simulink model "Parallel"  (R2020b)
settings: Solver=ode4  StartTime=0  StopTime=endtime  MaxStep=0.05  RelTol=1e-5
values from neighbouring files (symbols this model uses):
  Av = 1.545*1.805    (= 2.788725)    [InitiateParallel.m]
  Cd = 0.3    [InitiateParallel.m]
  Cr = 0.0032    [InitiateParallel.m]
  DCT = 1    [InitiateParallel.m]
  Density = (85*19.6e6 + 15*32e6)/100    (= 21460000)    [InitiateParallel.m]
  Eta_gen = 0.6    [InitiateParallel.m]
  EtaEM = Eta    [CreateEMmap.m]
  EtaGEAR = 0.97    [InitiateParallel.m]
  EtaICE = EtaICE_HeavyDIESEL    [InitiateParallel.m]
  EtaPE = 0.98    [InitiateParallel.m]
  grav = 9.81    [InitiateParallel.m]
  ksoc = max(Wbatt)/400/Tau_charge    [InitiateParallel.m]
  ksoc_vect = ksoc*tan(pi/2.05*[-1:1/15:1])*2    [InitiateParallel.m]
  Mv = 40000    [InitiateParallel.m]
  Number_of_gears = 12    [InitiateParallel.m]
  Paux = 3000    [InitiateParallel.m]
  Pem_max = 300000    [InitiateParallel.m]    (also in ParallelBatch_2D.m = EMpower_vector(loop2))
  Pice_max = 300000    [InitiateParallel.m]
  PtoT = zeros(length(P),4)    [CreateICEmap.m]
  rho_air = 1.2    [InitiateParallel.m]
  rw = 0.506    [InitiateParallel.m]
  SOC_batt_ref_value = 70    [InitiateParallel.m]
  SOC_batt_start_value = 100    [InitiateParallel.m]    (also in ParallelBatch_1D.m = SOC(length(SOC(:,1)),2))
  SOC_tract_max = 98    [InitiateParallel.m]
  SOC_tract_min = 12    [InitiateParallel.m]
  Tau_charge = 2    [InitiateParallel.m]
  Tem = Tem_max.*Tref/max(Tref)    [CreateEMmap.m]
  Tem_lim = min([Tem_max*ones(1,length(Wem)); Pem_max./Wem])    [CreateEMmap.m]
  Tem_max = Pem_max/(wice_max/fwr)    (= 2406.42273955)    [InitiateParallel.m]
  Tice_max = Pice_max/(wice_max*row/(length(EtaICE)-1))    [InitiateParallel.m]
  utvx_max = wice_max/((vmax/5)/rw)    (= 26.4940980453)    [InitiateParallel.m]
  Utvx_vect = zeros(1,Number_of_gears+1)    [InitiateParallel.m]
  Wbatt = 8.9*3.6e6    (= 32040000)    [InitiateParallel.m]
  Wem = wem_max.*w/max(w)    [CreateEMmap.m]
  wem_max = wice_max    (= 261.799387799)    [InitiateParallel.m]
  wice_max = 2500*2*pi/60    (= 261.799387799)    [InitiateParallel.m]
  wice_min = 700*2*pi/60    (= 73.3038285838)    [InitiateParallel.m]
undefined symbols (not defined in the file or in its folder): EtaBATT, FuelConsICE, Pbatt, Pbatt_max_new, Pice_max_parallel, Tice, Tlim_ice, Wice
libraries: simulink_need_slupdate x1, simulink x1
(part 1 of 2)
settings Model: ExtModeTrigMode=oneshot  ExtModeArmWhenConnect=off  Creator=Mats  LastModifiedBy=ielmats
settings DataIOCC: SaveFormat=Array  SignalLoggingSaveFormat=ModelDataLogs  ReturnWorkspaceOutputs=off  SignalLoggingName=sigsOut
settings OptimizationCC: BlockReduction=off  BooleanDataType=off  ExpressionDepthLimit=2147483647  InitFltsAndDblsToZero=on  LifeSpan=inf
settings DebuggingCC: ConsistencyChecking=warning  SaveWithParameterizedLinksMsg=none  UnderspecifiedInitializationDetection=Classic  MergeDetectMultiDrivingBlocksExec=none  SignalResolutionControl=TryResolveAllWithWarning  MultiTaskDSMMsg=warning  MultiTaskCondExecSysMsg=none  UnnecessaryDatatypeConvMsg=warning  FcnCallInpInsideContextMsg=warning  UnconnectedInputMsg=none  UnconnectedOutputMsg=none  UnconnectedLineMsg=none  StateNameClashWarn=warning  SFUnexpectedBacktrackingDiag=warning  SFNoUnconditionalDefaultTransitionDiag=warning  ArithmeticOperatorsInVariantConditions=warning
settings HardwareCC: ProdBitPerPointer=32  ProdBitPerSizeT=32  ProdBitPerPtrDiffT=32  ProdLargestAtomicFloat=None  ProdIntDivRoundTo=Undefined  ProdEndianess=Unspecified  ProdWordSize=32  ProdHWDeviceType=32-bit Generic  TargetHWDeviceType=32-bit Generic  TargetUnknown=on  ProdEqTarget=off
settings ModelReferenceCC: PropagateSignalLabelsOutOfModel=off
settings SFSimCC: SimUseLocalCustomCode=off  CustomCodeUndefinedFunction=UseInterfaceOnly
settings RTWCC: RTWUseLocalCustomCode=off
settings CodeAppCC: StateflowObjectComments=on
settings GRTTargetCC: TargetFcnLib=ansi_tfl_tmw.mat  TargetLangStandard=C89/C90 (ANSI)  CombineOutputUpdateFcns=off  GRTInterface=on
settings ConfigComp: CovMetricSettings=dw  CovSaveCumulativeToWorkspaceVar=on  CovSaveSingleToWorkspaceVar=on  CovExternalEMLEnable=off

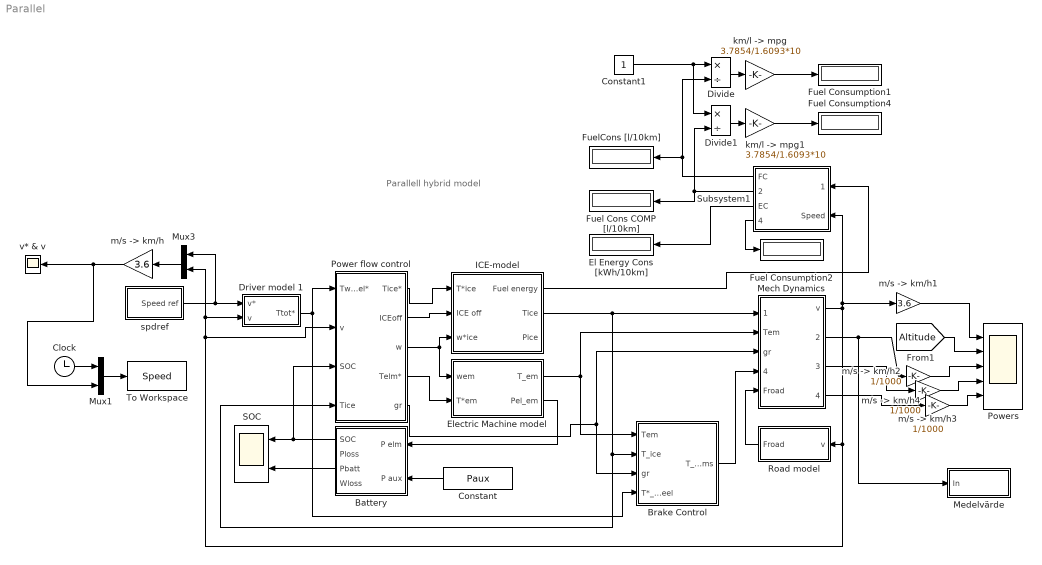
== system Parallel ==
  note: Parallell hybrid model
  Battery : Subsystem
  Brake Control : Subsystem
  Clock : Clock
  Constant : Constant  Value=Paux
  Constant1 : Constant
  Divide : Product  Inputs=*/
  Divide1 : Product  Inputs=*/
  Driver model 1 : Subsystem  mask{Mv=Mv, rw=rw, Pmax=Pice_max+Pem_max}
      mask prompts: Mv "Vehicle Mass"; rw "Wheel Radius"; Pmax "Max Wheel Power"
      mask init:
      | Ti = 2 + 1*(Mv-1000)/19000;
      | Kv=4*Mv/Ti;
  El Energy Cons [kWh/10km] : Display
  Electric Machine model : Subsystem
  Fuel Cons COMP [l/10km] : Display
  Fuel Consumption1 : Display
  Fuel Consumption2 : Display
  Fuel Consumption4 : Display
  FuelCons [l/10km] : Display
  ICE-model : Subsystem
  Mech Dynamics : Subsystem
  Medelvärde : Subsystem
  Mux1 : Mux  Inputs=2
  Mux3 : Mux  Inputs=2
  Power flow control : Subsystem
  Powers : Scope  NumInputPorts=5
  Road model : Subsystem
  SOC : Scope  NumInputPorts=2
  Subsystem1 : Subsystem
  To Workspace : ToWorkspace  VariableName=Speed  SampleTime=-1
  "km/l -> mpg" : Gain  Gain=3.7854/1.6093*10  SaturateOnIntegerOverflow=on  OutDataTypeStr=Inherit: Same as input  ParamDataTypeStr=Inherit: Same as input
  "km/l -> mpg1" : Gain  Gain=3.7854/1.6093*10  SaturateOnIntegerOverflow=on  OutDataTypeStr=Inherit: Same as input  ParamDataTypeStr=Inherit: Same as input
  "m/s -> km/h" : Gain  Gain=3.6  SaturateOnIntegerOverflow=on  OutDataTypeStr=Inherit: Same as input  ParamDataTypeStr=Inherit: Same as input
  "m/s -> km/h1" : Gain  Gain=3.6  SaturateOnIntegerOverflow=on  OutDataTypeStr=Inherit: Same as input  ParamDataTypeStr=Inherit: Same as input
  "m/s -> km/h2" : Gain  Gain=1/1000  SaturateOnIntegerOverflow=on  OutDataTypeStr=Inherit: Same as input  ParamDataTypeStr=Inherit: Same as input
  "m/s -> km/h3" : Gain  Gain=1/1000  SaturateOnIntegerOverflow=on  OutDataTypeStr=Inherit: Same as input  ParamDataTypeStr=Inherit: Same as input
  "m/s -> km/h4" : Gain  Gain=1/1000  SaturateOnIntegerOverflow=on  OutDataTypeStr=Inherit: Same as input  ParamDataTypeStr=Inherit: Same as input
  spdref : Subsystem
  v* & v : Scope
  wires:
  Power flow control/3(w) -> ICE-model/3(w*ice), Electric Machine model/1(wem)
  Constant/1 -> Battery/2(P aux)
  spdref/1(Speed ref) -> Driver model 1/1(v*), Mux3/1
  Driver model 1/1(Ttot*) -> Brake Control/4(T*_wheel), Power flow control/1(Twheel*)
  Mux3/1 -> "m/s -> km/h"/1
  Power flow control/5(gr) -> Brake Control/3(gr), Mech Dynamics/3(gr)
  Power flow control/4(Telm*) -> Electric Machine model/2(T*em)
  Power flow control/1(Tice*) -> ICE-model/1(T*ice)
  Mech Dynamics/1(v) -> Subsystem1/2(Speed), "m/s -> km/h1"/1, Driver model 1/2(v), Mux3/2, Power flow control/2(v), Road model/1("v ")
  Electric Machine model/1(T_em) -> Mech Dynamics/2(Tem), Brake Control/1(Tem)
  Electric Machine model/2(Pel_em) -> Battery/1(P elm)
  "m/s -> km/h"/1 -> Mux1/2, v* & v/1
  Battery/1(SOC) -> SOC/1, Power flow control/3(SOC)
  Power flow control/2(ICEoff) -> ICE-model/2(ICE off)
  Battery/3(Pbatt) -> SOC/2
  ICE-model/2(Tice) -> Power flow control/4(Tice), Brake Control/2(T_ice), Mech Dynamics/1(Tdrive)
  ICE-model/1(Fuel energy) -> Subsystem1/1(Fuel energy)
  [Altitude] -> Powers/2
  Mech Dynamics/2(Ptraction) -> Medelvärde/1(In), "m/s -> km/h2"/1
  Mech Dynamics/3(Pfriction) -> "m/s -> km/h3"/1
  Mech Dynamics/4(Pbrake) -> "m/s -> km/h4"/1
  "m/s -> km/h1"/1 -> Powers/1
  "m/s -> km/h2"/1 -> Powers/3
  "m/s -> km/h3"/1 -> Powers/4
  "m/s -> km/h4"/1 -> Powers/5
  Brake Control/1(T_broms) -> Mech Dynamics/4(Tbrake)
  Road model/1(Froad) -> Mech Dynamics/5(Froad)
  Subsystem1/4(dist (mil)) -> Fuel Consumption2/1
  Clock/1 -> Mux1/1
  Mux1/1 -> To Workspace/1
  Constant1/1 -> Divide1/1, Divide/1
  Divide/1 -> "km/l -> mpg"/1
  Subsystem1/1(FC) -> FuelCons [l/10km]/1, Divide/2
  Subsystem1/2(FCcomp) -> Divide1/2, Fuel Cons COMP [l/10km]/1
  Divide1/1 -> "km/l -> mpg1"/1
  "km/l -> mpg"/1 -> Fuel Consumption1/1
  "km/l -> mpg1"/1 -> Fuel Consumption4/1
  Subsystem1/3(EC) -> El Energy Cons [kWh/10km]/1

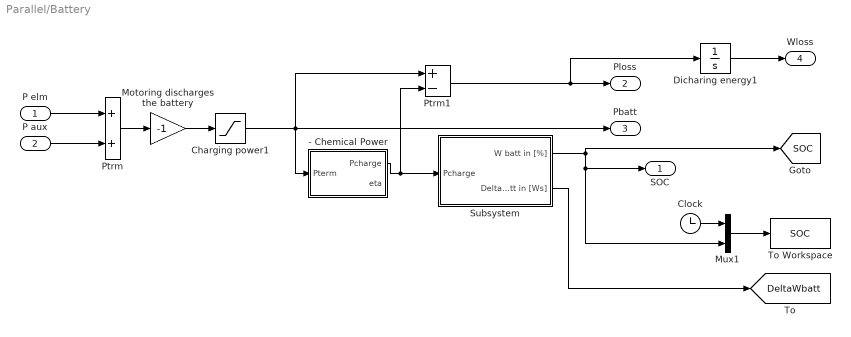
== system Parallel/Battery ==
  P elm : Inport
  P aux : Inport  Port=2
  - Chemical Power : Subsystem
  Charging power1 : Saturate  UpperLimit=Pbatt_max_new  LowerLimit=-Pbatt_max_new
  Clock : Clock
  Dicharing energy1 : Integrator  UpperSaturationLimit=-1
  Motoring discharges the battery : Gain  Gain=-1  SaturateOnIntegerOverflow=on  OutDataTypeStr=Inherit: Same as input  ParamDataTypeStr=Inherit: Same as input
  Mux1 : Mux  Inputs=2
  Ptrm : Sum  InputSameDT=on  SaturateOnIntegerOverflow=on  OutDataTypeStr=Inherit: Same as first input
  Ptrm1 : Sum  Inputs=+-  InputSameDT=on  SaturateOnIntegerOverflow=on  OutDataTypeStr=Inherit: Same as first input
  Subsystem : Subsystem
  To Workspace : ToWorkspace  VariableName=SOC  SampleTime=-1
  SOC : Outport  InitialOutput=0  VectorParamsAs1DForOutWhenUnconnected=off
  Ploss : Outport  Port=2  InitialOutput=0  VectorParamsAs1DForOutWhenUnconnected=off
  Pbatt : Outport  Port=3  InitialOutput=0  VectorParamsAs1DForOutWhenUnconnected=off
  Wloss : Outport  Port=4  InitialOutput=0  VectorParamsAs1DForOutWhenUnconnected=off
  tag scope: DeltaWbatt=global, SOC=global
  wires:
  P elm/1 -> Ptrm/1
  Ptrm/1 -> Motoring discharges the battery/1
  - Chemical Power/1(Pcharge) -> Ptrm1/2, Subsystem/1("Pcharge ")
  Ptrm1/1 -> Ploss/1, Dicharing energy1/1
  Motoring discharges the battery/1 -> Charging power1/1
  P aux/1 -> Ptrm/2
  Dicharing energy1/1 -> Wloss/1
  Charging power1/1 -> - Chemical Power/1(Pterm), Pbatt/1, Ptrm1/1
  Subsystem/1(W batt in [%]) -> Mux1/2, SOC/1, [SOC]
  Clock/1 -> Mux1/1
  Mux1/1 -> To Workspace/1
  Subsystem/2(DeltaWbatt in [Ws]) -> [DeltaWbatt]

== system Parallel/Brake Control ==
  note: If the drive train is not able
      | to supply the braking force, then
      | the friction brakes are used.
  Tem : Inport
  T_ice : Inport  Port=2
  gr : Inport  Port=3
  T*_wheel : Inport  Port=4
  -> hjulmoment : Product  InputSameDT=on  SaturateOnIntegerOverflow=on  OutDataTypeStr=Inherit: Same as first input
  Endast negativa bromsmoment1 : Saturate  UpperLimit=0  LowerLimit=-inf
  Mux : Mux  Inputs=2
  Scope : Scope
  Sum1 : Sum  Inputs=-+  InputSameDT=on  SaturateOnIntegerOverflow=on  OutDataTypeStr=Inherit: Same as first input
  Sum2 : Sum  InputSameDT=on  SaturateOnIntegerOverflow=on  OutDataTypeStr=Inherit: Same as first input
  T_broms : Outport  InitialOutput=0  VectorParamsAs1DForOutWhenUnconnected=off
  wires:
  Tem/1 -> Sum2/1
  T_ice/1 -> Sum2/2
  Sum2/1 -> -> hjulmoment/1
  gr/1 -> -> hjulmoment/2
  -> hjulmoment/1 -> Mux/1, Sum1/1
  T*_wheel/1 -> Sum1/2, Mux/2
  Sum1/1 -> Endast negativa bromsmoment1/1
  Endast negativa bromsmoment1/1 -> T_broms/1
  Mux/1 -> Scope/1

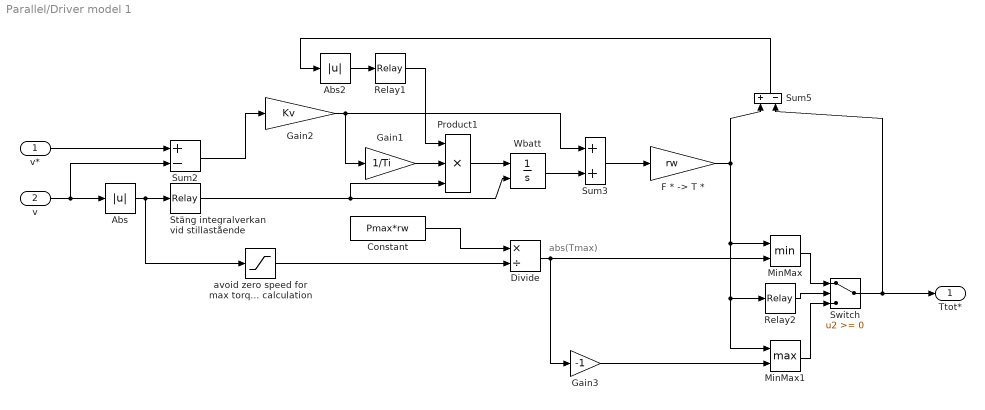
== system Parallel/Driver model 1 ==
  note: abs(Tmax)
  v* : Inport
  v : Inport  Port=2
  Abs : Abs  SaturateOnIntegerOverflow=on
  Abs2 : Abs  SaturateOnIntegerOverflow=on
  Constant : Constant  Value=Pmax*rw
  Divide : Product  Inputs=*/
  "F * -> T *" : Gain  Gain=rw  SaturateOnIntegerOverflow=on  OutDataTypeStr=Inherit: Same as input  ParamDataTypeStr=Inherit: Same as input
  Gain1 : Gain  Gain=1/Ti  SaturateOnIntegerOverflow=on  OutDataTypeStr=Inherit: Same as input  ParamDataTypeStr=Inherit: Same as input
  Gain2 : Gain  Gain=Kv  SaturateOnIntegerOverflow=on  OutDataTypeStr=Inherit: Same as input  ParamDataTypeStr=Inherit: Same as input
  Gain3 : Gain  Gain=-1  SaturateOnIntegerOverflow=on  OutDataTypeStr=Inherit: Same as input  ParamDataTypeStr=Inherit: Same as input
  MinMax : MinMax  Inputs=2
  MinMax1 : MinMax  Function=max  Inputs=2
  Product1 : Product  Inputs=3  InputSameDT=on  SaturateOnIntegerOverflow=on  OutDataTypeStr=Inherit: Same as first input
  Relay1 : Relay  OnOutputValue=0  OffOutputValue=1
  Relay2 : Relay  OnOutputValue=10  OffOutputValue=1
  Stäng integralverkan vid stillastående : Relay  OnSwitchValue=0.3  OffSwitchValue=0.3-eps
  Sum2 : Sum  Inputs=+-  InputSameDT=on  SaturateOnIntegerOverflow=on  OutDataTypeStr=Inherit: Same as first input
  Sum3 : Sum  InputSameDT=on  SaturateOnIntegerOverflow=on  OutDataTypeStr=Inherit: Same as first input
  Sum5 : Sum  Inputs=+-  InputSameDT=on  SaturateOnIntegerOverflow=on  OutDataTypeStr=Inherit: Same as first input
  Switch : Switch
  Wbatt : Integrator  ExternalReset=falling  UpperSaturationLimit=10000  LowerSaturationLimit=-100000
  avoid zero speed for max torque calculation : Saturate  UpperLimit=inf  LowerLimit=5/3.6
  Ttot* : Outport  InitialOutput=0  VectorParamsAs1DForOutWhenUnconnected=off
  wires:
  Sum5/1 -> Abs2/1
  Relay1/1 -> Product1/1
  Abs2/1 -> Relay1/1
  Gain1/1 -> Product1/2
  Abs/1 -> Stäng integralverkan vid stillastående/1, avoid zero speed for max torque calculation/1
  Product1/1 -> Wbatt/1
  Sum3/1 -> "F * -> T *"/1
  Wbatt/1 -> Sum3/2
  "F * -> T *"/1 -> MinMax/1, MinMax1/1, Relay2/1, Sum5/1
  Gain2/1 -> Gain1/1, Sum3/1
  Stäng integralverkan vid stillastående/1 -> Product1/3, Wbatt/2
  Sum2/1 -> Gain2/1
  v*/1 -> Sum2/1
  v/1 -> Abs/1, Sum2/2
  Constant/1 -> Divide/1
  avoid zero speed for max torque calculation/1 -> Divide/2
  Divide/1 -> Gain3/1, MinMax/2
  Gain3/1 -> MinMax1/2
  Relay2/1 -> Switch/2
  MinMax/1 -> Switch/1
  MinMax1/1 -> Switch/3
  Switch/1 -> Ttot*/1, Sum5/2

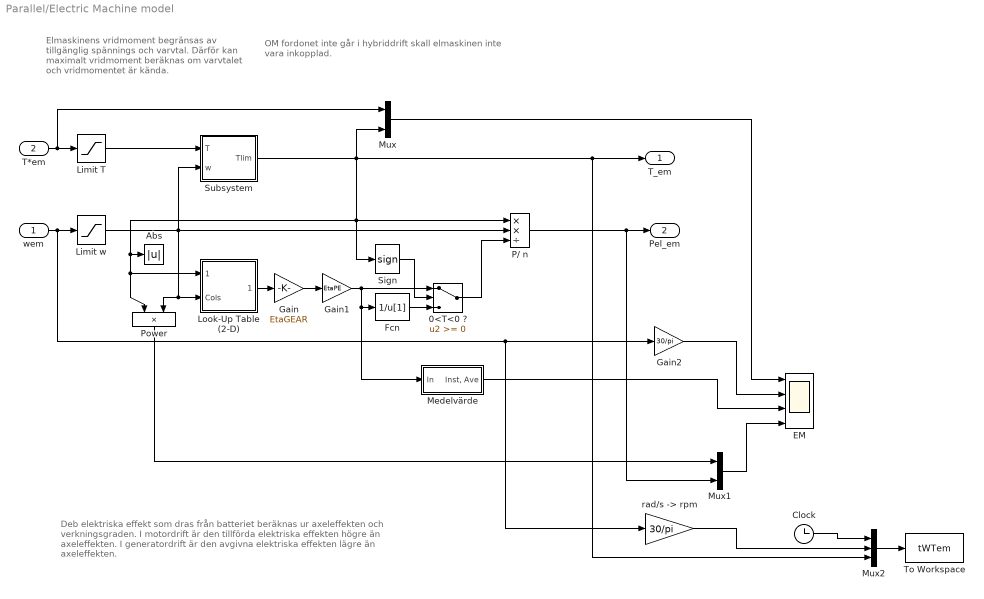
== system Parallel/Electric Machine model ==
  note: Elmaskinens vridmoment begränsas
      | av tillgänglig spännings och varvtal. Därför
      | kan maximalt vridmoment beräknas
      | om varvtalet och vridmomentet är kända.
  note: OM fordonet inte går i hybriddrift skall elmaskinen inte
      | vara inkopplad.
  note: Deb elektriska effekt som dras från batteriet beräknas ur axeleffekten
      | och verkningsgraden. I motordrift är den tillförda elektriska effekten
      | högre än axeleffekten. I generatordrift är den avgivna elektriska effekten
      | lägre än axeleffekten.
  wem : Inport
  T*em : Inport  Port=2
  0<T<0 ? : Switch  SaturateOnIntegerOverflow=on  InputSameDT=on
  Abs : Abs  SaturateOnIntegerOverflow=on
  Clock : Clock
  EM : Scope  NumInputPorts=4
  Fcn : Fcn  Expr=1/u[1]
  Gain : Gain  Gain=EtaGEAR  SaturateOnIntegerOverflow=on  OutDataTypeStr=Inherit: Same as input  ParamDataTypeStr=Inherit: Same as input
  Gain1 : Gain  Gain=EtaPE  SaturateOnIntegerOverflow=on  OutDataTypeStr=Inherit: Same as input  ParamDataTypeStr=Inherit: Same as input
  Gain2 : Gain  Gain=30/pi  SaturateOnIntegerOverflow=on  OutDataTypeStr=Inherit: Same as input  ParamDataTypeStr=Inherit: Same as input
  Limit T : Saturate  UpperLimit=Tem_max  LowerLimit=-Tem_max
  Limit w : Saturate  UpperLimit=wem_max  LowerLimit=0
  Look-Up Table (2-D) : Subsystem  mask(Lookup Table (2-D)){x=Tem, y=Wem, t=EtaEM}
      mask prompts: x "Row:"; y "Column:"; t "Table:"
      mask help: Performs 2-D linear interpolation of input values using the specified input/output table. Extrapolation is performed outside the table boundaries. The first dimension corresponds to the top (or left) input port.
      mask init:
      | [r,c]=size(t);
      | xt=reshape(x,prod(size(x)),1);
      | xi=xt(:,ones(1,c));
      | minx=min(x); maxx=max(x);
      | mint=min(min(t)); maxt=max(max(t));
      mask Display: plot(double(xi),double(t),double([minx maxx]),double([mint mint]),double([minx minx]),double([mint maxt]))
  Medelvärde : Subsystem
  Mux : Mux  Inputs=2
  Mux1 : Mux  Inputs=2
  Mux2 : Mux  Inputs=3
  P/ n : Product  Inputs=**/  InputSameDT=on  SaturateOnIntegerOverflow=on  OutDataTypeStr=Inherit: Same as first input
  Power : Product  SaturateOnIntegerOverflow=on  OutDataTypeStr=Inherit: Same as first input
  Sign : Signum
  Subsystem : Subsystem  mask{Tmax=Tem_max, Pmax=Pem_max}
      mask prompts: Tmax "Max Torque"; Pmax "Max Power"
      mask Display:
      | plot(-120,-120,120,120)
      | plot([-110 110],[0 0],[0 0],[-110 110])
      | plot([-20 20],[90 90],[-20 20],[-90 -90])
      | 
      | plot([-100 :-20],-90*20./[-100:-20])
      | plot([-100 :-20],90*20./[-100:-20])
      | plot([20:100],-90*20./[20:100])
      | plot([20:100],90*20./[20:100])
  To Workspace : ToWorkspace  VariableName=tWTem  SampleTime=-1
  "rad/s -> rpm" : Gain  Gain=30/pi  SaturateOnIntegerOverflow=on  OutDataTypeStr=Inherit: Same as input  ParamDataTypeStr=Inherit: Same as input
  T_em : Outport  InitialOutput=0  VectorParamsAs1DForOutWhenUnconnected=off
  Pel_em : Outport  Port=2  InitialOutput=0  VectorParamsAs1DForOutWhenUnconnected=off
  wires:
  wem/1 -> Limit w/1, Gain2/1, "rad/s -> rpm"/1
  Sign/1 -> 0<T<0 ?/2
  P/ n/1 -> Pel_em/1, Mux1/2
  T*em/1 -> Limit T/1, Mux/1
  Fcn/1 -> 0<T<0 ?/3
  Look-Up Table (2-D)/1(Out1) -> Gain/1
  Limit T/1 -> Subsystem/1(T)
  Limit w/1 -> Look-Up Table (2-D)/2(Cols), Power/2, P/ n/2, Subsystem/2(w)
  Medelvärde/1("Inst, Ave") -> EM/3
  Mux/1 -> EM/1
  Power/1 -> Mux1/1
  Mux1/1 -> EM/4
  Gain/1 -> Gain1/1
  Gain1/1 -> 0<T<0 ?/1, Medelvärde/1(In), Fcn/1
  Subsystem/1(Tlim) -> Mux/2, Power/1, Look-Up Table (2-D)/1(Rows), Abs/1, Sign/1, P/ n/1, T_em/1, Mux2/3
  0<T<0 ?/1 -> P/ n/3
  "rad/s -> rpm"/1 -> Mux2/2
  Clock/1 -> Mux2/1
  Mux2/1 -> To Workspace/1
  Gain2/1 -> EM/2

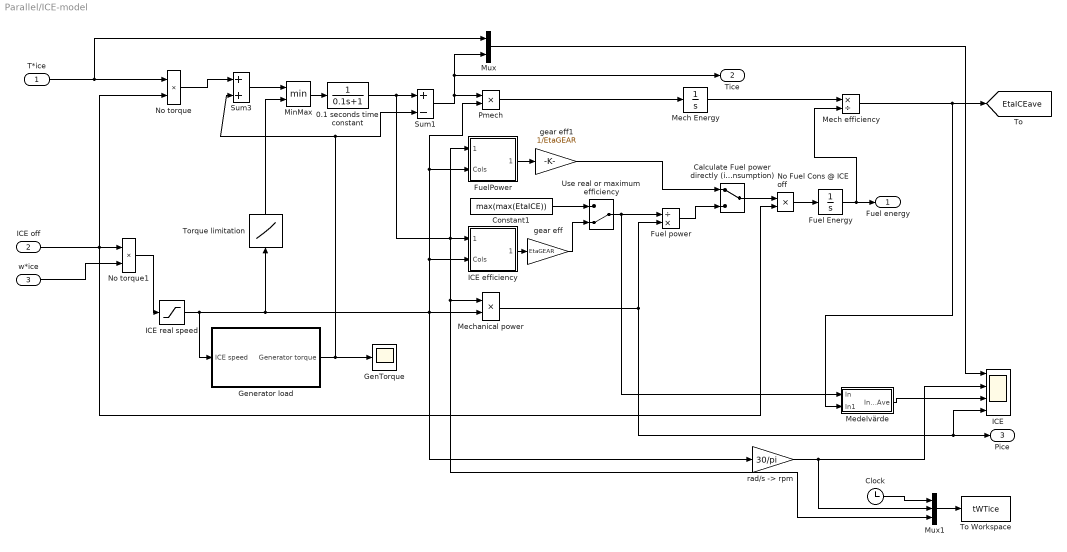
== system Parallel/ICE-model ==
  T*ice : Inport
  ICE off : Inport  Port=2
  w*ice : Inport  Port=3
  0.1 seconds time constant : TransferFcn  Denominator=[0.1 1]
  Calculate Fuel power directly (including idle consumption) : ManualSwitch
  Clock : Clock
  Constant1 : Constant  Value=max(max(EtaICE))
  Fuel Energy : Integrator
  Fuel power : Product  Inputs=/*  InputSameDT=on  SaturateOnIntegerOverflow=on  OutDataTypeStr=Inherit: Same as first input
  FuelPower : Subsystem  mask(Lookup Table (2-D)){x=Tice, y=Wice, t=FuelConsICE}
      mask prompts: x "Row:"; y "Column:"; t "Table:"
      mask help: Performs 2-D linear interpolation of input values using the specified input/output table. Extrapolation is performed outside the table boundaries. The first dimension corresponds to the top (or left) input port.
      mask init:
      | [r,c]=size(t);
      | xt=reshape(x,prod(size(x)),1);
      | xi=xt(:,ones(1,c));
      | minx=min(x); maxx=max(x);
      | mint=min(min(t)); maxt=max(max(t));
      mask Display: plot(double(xi),double(t),double([minx maxx]),double([mint mint]),double([minx minx]),double([mint maxt]))
  GenTorque : Scope
  Generator load : Subsystem
  ICE : Scope  NumInputPorts=4
  ICE efficiency : Subsystem  mask(Lookup Table (2-D)){x=Tice, y=Wice, t=EtaICE}
      mask prompts: x "Row:"; y "Column:"; t "Table:"
      mask help: Performs 2-D linear interpolation of input values using the specified input/output table. Extrapolation is performed outside the table boundaries. The first dimension corresponds to the top (or left) input port.
      mask init:
      | [r,c]=size(t);
      | xt=reshape(x,prod(size(x)),1);
      | xi=xt(:,ones(1,c));
      | minx=min(x); maxx=max(x);
      | mint=min(min(t)); maxt=max(max(t));
      mask Display: plot(double(xi),double(t),double([minx maxx]),double([mint mint]),double([minx minx]),double([mint maxt]))
  ICE real speed : Saturate  UpperLimit=wice_max  LowerLimit=wice_min
  Mech Energy : Integrator
  Mech efficiency : Product  Inputs=*/  InputSameDT=on  SaturateOnIntegerOverflow=on  OutDataTypeStr=Inherit: Same as first input
  Mechanical power : Product  InputSameDT=on  SaturateOnIntegerOverflow=on  OutDataTypeStr=Inherit: Same as first input
  Medelvärde : Subsystem
  MinMax : MinMax  Inputs=2  InputSameDT=on  SaturateOnIntegerOverflow=on
  Mux : Mux  Inputs=2
  Mux1 : Mux  Inputs=3
  No Fuel Cons @ ICE off : Product  Inputs=**  InputSameDT=on  SaturateOnIntegerOverflow=on  OutDataTypeStr=Inherit: Same as first input
  No torque : Product  SaturateOnIntegerOverflow=on  OutDataTypeStr=Inherit: Same as first input
  No torque1 : Product  SaturateOnIntegerOverflow=on  OutDataTypeStr=Inherit: Same as first input
  Pmech : Product  Inputs=**  InputSameDT=on  SaturateOnIntegerOverflow=on  OutDataTypeStr=Inherit: Same as first input
  Sum1 : Sum  Inputs=+-  SaturateOnIntegerOverflow=on
  Sum3 : Sum  SaturateOnIntegerOverflow=on
  To Workspace : ToWorkspace  VariableName=tWTice  SampleTime=-1
  Torque limitation : Lookup  InputValues=Wice  Table=Tlim_ice  SaturateOnIntegerOverflow=on
  Use real or maximum efficiency : ManualSwitch  CurrentSetting=0
  gear eff : Gain  Gain=EtaGEAR  SaturateOnIntegerOverflow=on  OutDataTypeStr=Inherit: Same as input  ParamDataTypeStr=Inherit: Same as input
  gear eff1 : Gain  Gain=1/EtaGEAR  SaturateOnIntegerOverflow=on  OutDataTypeStr=Inherit: Same as input  ParamDataTypeStr=Inherit: Same as input
  "rad/s -> rpm" : Gain  Gain=30/pi  SaturateOnIntegerOverflow=on  OutDataTypeStr=Inherit: Same as input  ParamDataTypeStr=Inherit: Same as input
  Fuel energy : Outport  InitialOutput=0  VectorParamsAs1DForOutWhenUnconnected=off
  Tice : Outport  Port=2  InitialOutput=0  VectorParamsAs1DForOutWhenUnconnected=off
  Pice : Outport  Port=3  InitialOutput=0  VectorParamsAs1DForOutWhenUnconnected=off
  tag scope: EtaICEave=global
  wires:
  Mux/1 -> ICE/1
  MinMax/1 -> 0.1 seconds time constant/1
  Torque limitation/1 -> MinMax/2
  Medelvärde/1("Inst, Ave") -> ICE/3
  "rad/s -> rpm"/1 -> ICE/2, Mux1/2
  Fuel Energy/1 -> Mech efficiency/2, Fuel energy/1
  ICE efficiency/1(Out1) -> gear eff/1
  Clock/1 -> Mux1/1
  Mux1/1 -> To Workspace/1
  Mechanical power/1 -> Fuel power/2, Pice/1, ICE/4
  Generator load/1(Generator torque) -> GenTorque/1, Sum3/2, Sum1/2
  Sum1/1 -> Tice/1, Mux/2, Pmech/1
  Sum3/1 -> MinMax/1
  0.1 seconds time constant/1 -> Sum1/1, ICE efficiency/1(Rows), Mechanical power/1, Mux1/3, FuelPower/1(Rows)
  Fuel power/1 -> Calculate Fuel power directly (including idle consumption)/2
  FuelPower/1(Out1) -> gear eff1/1
  gear eff1/1 -> Calculate Fuel power directly (including idle consumption)/1
  Constant1/1 -> Use real or maximum efficiency/1
  gear eff/1 -> Use real or maximum efficiency/2
  Use real or maximum efficiency/1 -> Medelvärde/1(In), Fuel power/1
  ICE real speed/1 -> Generator load/1(ICE speed), Torque limitation/1, Pmech/2, FuelPower/2(Cols), ICE efficiency/2(Cols), Mechanical power/2, "rad/s -> rpm"/1
  T*ice/1 -> Mux/1, No torque/1
  No torque/1 -> Sum3/1
  No torque1/1 -> ICE real speed/1
  ICE off/1 -> No torque1/1, No torque/2, No Fuel Cons @ ICE off/2
  Calculate Fuel power directly (including idle consumption)/1 -> No Fuel Cons @ ICE off/1
  No Fuel Cons @ ICE off/1 -> Fuel Energy/1
  w*ice/1 -> No torque1/2
  Pmech/1 -> Mech Energy/1
  Mech Energy/1 -> Mech efficiency/1
  Mech efficiency/1 -> [EtaICEave], Medelvärde/2(In1)

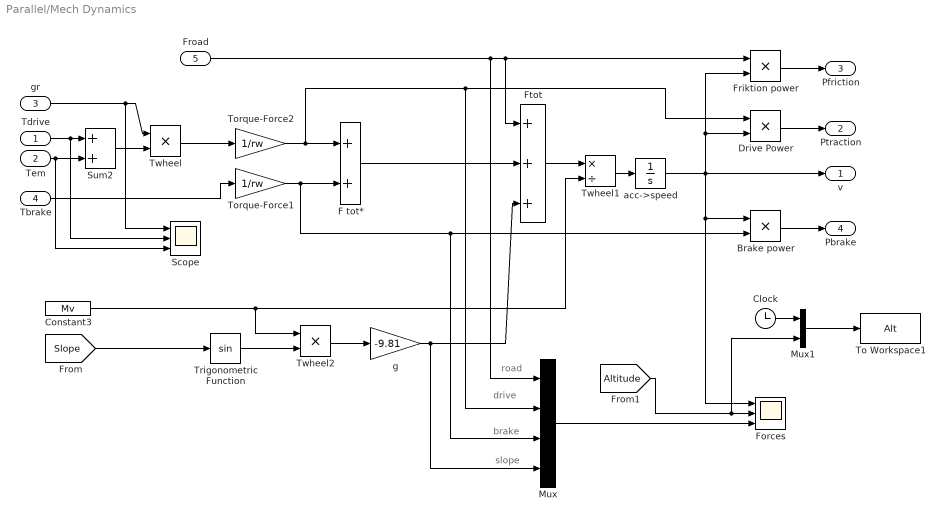
== system Parallel/Mech Dynamics ==
  note: road
  note: drive
  note: brake
  note: slope
  Tdrive : Inport
  Tem : Inport  Port=2
  gr : Inport  Port=3
  Tbrake : Inport  Port=4
  Froad : Inport  Port=5
  Brake power : Product  InputSameDT=on  SaturateOnIntegerOverflow=on  OutDataTypeStr=Inherit: Same as first input
  Clock : Clock
  Constant3 : Constant  Value=Mv
  Drive Power : Product  InputSameDT=on  SaturateOnIntegerOverflow=on  OutDataTypeStr=Inherit: Same as first input
  F tot* : Sum  InputSameDT=on  SaturateOnIntegerOverflow=on  OutDataTypeStr=Inherit: Same as first input
  Forces : Scope  NumInputPorts=3
  Friktion power : Product  InputSameDT=on  SaturateOnIntegerOverflow=on  OutDataTypeStr=Inherit: Same as first input
  Ftot : Sum  Inputs=+++  InputSameDT=on  SaturateOnIntegerOverflow=on  OutDataTypeStr=Inherit: Same as first input
  Mux : Mux
  Mux1 : Mux  Inputs=2
  Scope : Scope  NumInputPorts=3
  Sum2 : Sum  InputSameDT=on  SaturateOnIntegerOverflow=on  OutDataTypeStr=Inherit: Same as first input
  To Workspace1 : ToWorkspace  VariableName=Alt  SampleTime=-1
  Torque-Force1 : Gain  Gain=1/rw  SaturateOnIntegerOverflow=on  OutDataTypeStr=Inherit: Same as input  ParamDataTypeStr=Inherit: Same as input
  Torque-Force2 : Gain  Gain=1/rw  SaturateOnIntegerOverflow=on  OutDataTypeStr=Inherit: Same as input  ParamDataTypeStr=Inherit: Same as input
  Trigonometric Function : Trigonometry
  Twheel : Product  InputSameDT=on  SaturateOnIntegerOverflow=on  OutDataTypeStr=Inherit: Same as first input
  Twheel1 : Product  Inputs=*/  InputSameDT=on  SaturateOnIntegerOverflow=on  OutDataTypeStr=Inherit: Same as first input
  Twheel2 : Product  Inputs=**  InputSameDT=on  SaturateOnIntegerOverflow=on  OutDataTypeStr=Inherit: Same as first input
  acc->speed : Integrator  LimitOutput=on  LowerSaturationLimit=0
  g : Gain  Gain=-9.81  SaturateOnIntegerOverflow=on  OutDataTypeStr=Inherit: Same as input  ParamDataTypeStr=Inherit: Same as input
  v : Outport  InitialOutput=0  VectorParamsAs1DForOutWhenUnconnected=off
  Ptraction : Outport  Port=2  InitialOutput=0  VectorParamsAs1DForOutWhenUnconnected=off
  Pfriction : Outport  Port=3  InitialOutput=0  VectorParamsAs1DForOutWhenUnconnected=off
  Pbrake : Outport  Port=4  InitialOutput=0  VectorParamsAs1DForOutWhenUnconnected=off
  wires:
  Twheel1/1 -> acc->speed/1
  acc->speed/1 -> Friktion power/2, Drive Power/2, Brake power/1, Forces/1, v/1
  Tbrake/1 -> Torque-Force1/1
  F tot*/1 -> Ftot/2
  Ftot/1 -> Twheel1/1
  Froad/1 -> Ftot/1, Friktion power/1, Mux/1
  Friktion power/1 -> Pfriction/1
  Constant3/1 -> Twheel1/2, Twheel2/1
  Trigonometric Function/1 -> Twheel2/2
  Twheel2/1 -> g/1
  g/1 -> Ftot/3, Mux/4
  [Slope] -> Trigonometric Function/1
  [Altitude] -> Mux1/2, Forces/2
  Mux/1 -> Forces/3
  Drive Power/1 -> Ptraction/1
  Torque-Force1/1 -> F tot*/2, Brake power/2, Mux/3
  Torque-Force2/1 -> F tot*/1, Drive Power/1, Mux/2
  Brake power/1 -> Pbrake/1
  Twheel/1 -> Torque-Force2/1
  gr/1 -> Twheel/1, Scope/1
  Tem/1 -> Sum2/2, Scope/3
  Tdrive/1 -> Sum2/1, Scope/2
  Sum2/1 -> Twheel/2
  Clock/1 -> Mux1/1
  Mux1/1 -> To Workspace1/1

== system Parallel/Medelvärde ==
  note: Denna del "mäter" tiden då motorn
      | är till, d.v.s. då verkningsgraden är
      | större än 1 %. Om den är 5 % antas
      | motorn stå still.
  In : Inport
  Integral : Integrator
  Integral1 : Integrator  InitialCondition=eps  LimitOutput=on  LowerSaturationLimit=eps
  Medelv : Product  Inputs=*/  InputSameDT=on  SaturateOnIntegerOverflow=on  OutDataTypeStr=Inherit: Same as first input
  Medelv1 : Product  Inputs=**  InputSameDT=on  SaturateOnIntegerOverflow=on  OutDataTypeStr=Inherit: Same as first input
  Mux : Mux  Inputs=2
  Relay : Relay  OnSwitchValue=0.05  OffSwitchValue=0.04
  Scope : Scope
  wires:
  Mux/1 -> Scope/1
  Medelv/1 -> Mux/2
  Relay/1 -> Integral1/1, Medelv1/2
  In/1 -> Relay/1, Medelv1/1, Mux/1
  Integral/1 -> Medelv/1
  Integral1/1 -> Medelv/2
  Medelv1/1 -> Integral/1

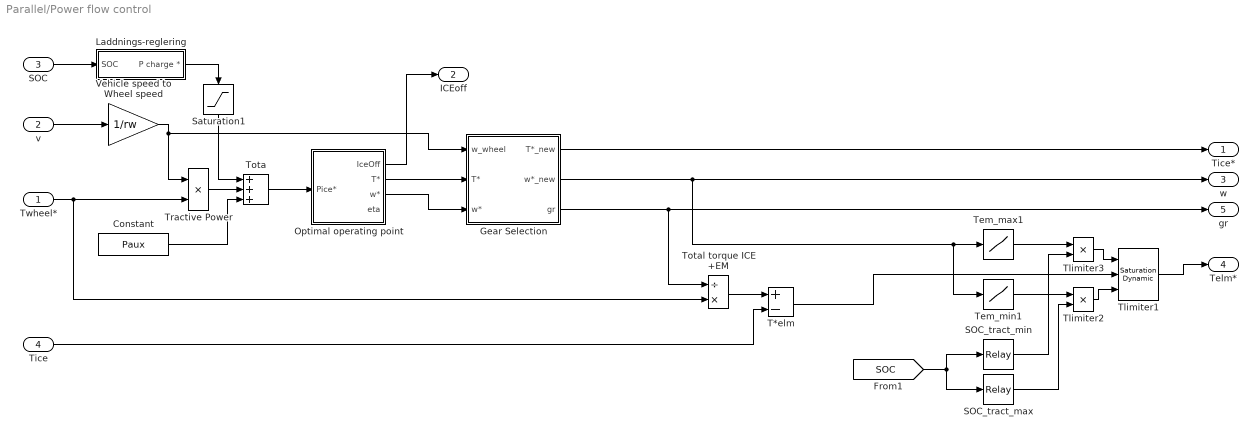
== system Parallel/Power flow control ==
  Twheel* : Inport
  v : Inport  Port=2
  SOC : Inport  Port=3
  Tice : Inport  Port=4
  Constant : Constant  Value=Paux
  Gear Selection : Subsystem
  Laddnings-reglering : Subsystem
  Optimal operating point : Subsystem
  SOC_tract_max : Relay  OnSwitchValue=SOC_tract_max+1  OffSwitchValue=SOC_tract_max-1  OnOutputValue=0  OffOutputValue=1
  SOC_tract_min : Relay  OnSwitchValue=SOC_tract_min+1  OffSwitchValue=SOC_tract_min-1
  Saturation1 : Saturate  UpperLimit=Pem_max  LowerLimit=-Pem_max
  T*elm : Sum  Inputs=+-  InputSameDT=on  SaturateOnIntegerOverflow=on  OutDataTypeStr=Inherit: Same as first input
  Tem_max1 : Lookup  InputValues=Wem  Table=Tem_lim  SaturateOnIntegerOverflow=on
  Tem_min1 : Lookup  InputValues=Wem  Table=-Tem_lim  SaturateOnIntegerOverflow=on
  Tlimiter1 : simulink/Discontinuities/Saturation Dynamic  OutMin=[]  OutMax=[]  OutDataTypeStr=Inherit: Same as second input  OutDataType=fixdt(1, 16)  OutScaling=2^-10  DoSatur=off
  Tlimiter2 : Product  Inputs=**  InputSameDT=on  SaturateOnIntegerOverflow=on  OutDataTypeStr=Inherit: Same as first input
  Tlimiter3 : Product  Inputs=**  InputSameDT=on  SaturateOnIntegerOverflow=on  OutDataTypeStr=Inherit: Same as first input
  Tota : Sum  Inputs=+++  InputSameDT=on  SaturateOnIntegerOverflow=on  OutDataTypeStr=Inherit: Same as first input
  Total torque ICE +EM : Product  Inputs=/*  InputSameDT=on  SaturateOnIntegerOverflow=on  OutDataTypeStr=Inherit: Same as first input
  Tractive Power : Product  InputSameDT=on  SaturateOnIntegerOverflow=on  OutDataTypeStr=Inherit: Same as first input
  Vehicle speed to Wheel speed : Gain  Gain=1/rw  SaturateOnIntegerOverflow=on  OutDataTypeStr=Inherit: Same as input  ParamDataTypeStr=Inherit: Same as input
  Tice* : Outport  VectorParamsAs1DForOutWhenUnconnected=off
  ICEoff : Outport  Port=2  VectorParamsAs1DForOutWhenUnconnected=off
  w : Outport  Port=3  VectorParamsAs1DForOutWhenUnconnected=off
  Telm* : Outport  Port=4  VectorParamsAs1DForOutWhenUnconnected=off
  gr : Outport  Port=5  VectorParamsAs1DForOutWhenUnconnected=off
  wires:
  Vehicle speed to Wheel speed/1 -> Tractive Power/1, Gear Selection/1(w_wheel)
  Twheel*/1 -> Tractive Power/2, Total torque ICE +EM/2
  v/1 -> Vehicle speed to Wheel speed/1
  Gear Selection/3(gr) -> Total torque ICE +EM/1, gr/1
  Optimal operating point/3(w*) -> Gear Selection/3(w*)
  Optimal operating point/2(T*) -> Gear Selection/2(T*)
  SOC/1 -> Laddnings-reglering/1(SOC)
  Tractive Power/1 -> Tota/2
  Tota/1 -> Optimal operating point/1(Pice*)
  T*elm/1 -> Tlimiter1/2
  Tice/1 -> T*elm/2
  Total torque ICE +EM/1 -> T*elm/1
  Gear Selection/1(T*_new) -> Tice*/1
  Gear Selection/2(w*_new) -> Tem_min1/1, Tem_max1/1, w/1
  Laddnings-reglering/1(P charge *) -> Saturation1/1
  [SOC] -> SOC_tract_max/1, SOC_tract_min/1
  Tem_max1/1 -> Tlimiter3/1
  Tlimiter3/1 -> Tlimiter1/1
  Tem_min1/1 -> Tlimiter2/1
  Tlimiter2/1 -> Tlimiter1/3
  SOC_tract_min/1 -> Tlimiter3/2
  SOC_tract_max/1 -> Tlimiter2/2
  Saturation1/1 -> Tota/1
  Constant/1 -> Tota/3
  Optimal operating point/1(IceOff) -> ICEoff/1
  Tlimiter1/1 -> Telm*/1

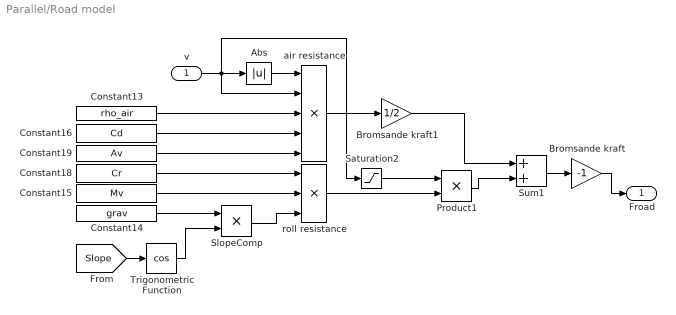
== system Parallel/Road model ==
  "v " : Inport
  Abs : Abs  SaturateOnIntegerOverflow=on
  Bromsande kraft : Gain  Gain=-1  SaturateOnIntegerOverflow=on  OutDataTypeStr=Inherit: Same as input  ParamDataTypeStr=Inherit: Same as input
  Bromsande kraft1 : Gain  Gain=1/2  SaturateOnIntegerOverflow=on  OutDataTypeStr=Inherit: Same as input  ParamDataTypeStr=Inherit: Same as input
  Constant13 : Constant  Value=rho_air
  Constant14 : Constant  Value=grav
  Constant15 : Constant  Value=Mv
  Constant16 : Constant  Value=Cd
  Constant18 : Constant  Value=Cr
  Constant19 : Constant  Value=Av
  Product1 : Product  InputSameDT=on  SaturateOnIntegerOverflow=on  OutDataTypeStr=Inherit: Same as first input
  Saturation2 : Saturate  UpperLimit=1  LowerLimit=-1
  SlopeComp : Product  Inputs=**  InputSameDT=on  SaturateOnIntegerOverflow=on  OutDataTypeStr=Inherit: Same as first input
  Sum1 : Sum  InputSameDT=on  SaturateOnIntegerOverflow=on  OutDataTypeStr=Inherit: Same as first input
  Trigonometric Function : Trigonometry  Operator=cos
  air resistance : Product  Inputs=5  InputSameDT=on  SaturateOnIntegerOverflow=on  OutDataTypeStr=Inherit: Same as first input
  roll resistance : Product  Inputs=3  InputSameDT=on  SaturateOnIntegerOverflow=on  OutDataTypeStr=Inherit: Same as first input
  Froad : Outport  InitialOutput=0  VectorParamsAs1DForOutWhenUnconnected=off
  wires:
  Abs/1 -> air resistance/1
  Constant15/1 -> roll resistance/2
  Constant18/1 -> roll resistance/1
  Constant19/1 -> air resistance/5
  Constant16/1 -> air resistance/4
  Constant13/1 -> air resistance/3
  Product1/1 -> Sum1/2
  air resistance/1 -> Bromsande kraft1/1
  Saturation2/1 -> Product1/1
  Sum1/1 -> Bromsande kraft/1
  "v "/1 -> Abs/1, Saturation2/1, air resistance/2
  Bromsande kraft/1 -> Froad/1
  Bromsande kraft1/1 -> Sum1/1
  roll resistance/1 -> Product1/2
  Trigonometric Function/1 -> SlopeComp/2
  [Slope] -> Trigonometric Function/1
  Constant14/1 -> SlopeComp/1
  SlopeComp/1 -> roll resistance/3

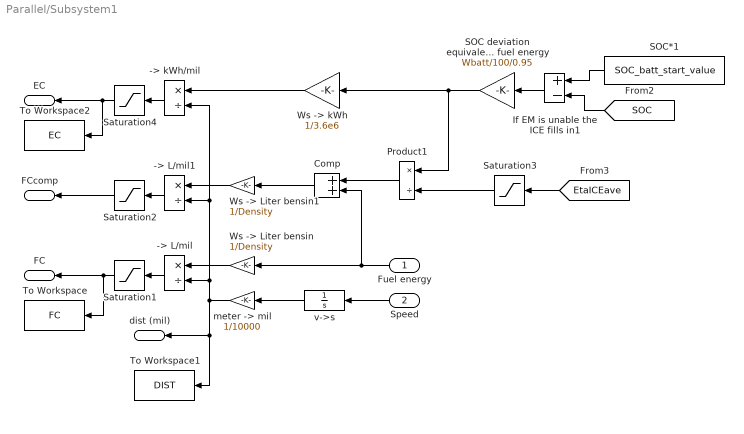
== system Parallel/Subsystem1 ==
  Fuel energy : Inport
  Speed : Inport  Port=2
  -> L/mil : Product  Inputs=*/  InputSameDT=on  SaturateOnIntegerOverflow=on  OutDataTypeStr=Inherit: Same as first input
  -> L/mil1 : Product  Inputs=*/  InputSameDT=on  SaturateOnIntegerOverflow=on  OutDataTypeStr=Inherit: Same as first input
  -> kWh/mil : Product  Inputs=*/  InputSameDT=on  SaturateOnIntegerOverflow=on  OutDataTypeStr=Inherit: Same as first input
  Comp : Sum  InputSameDT=on  SaturateOnIntegerOverflow=on  OutDataTypeStr=Inherit: Same as first input
  If EM is unable the ICE fills in1 : Sum  Inputs=+-  InputSameDT=on  SaturateOnIntegerOverflow=on  OutDataTypeStr=Inherit: Same as first input
  Product1 : Product  Inputs=*/  SaturateOnIntegerOverflow=on  OutDataTypeStr=Inherit: Same as first input
  SOC deviation equivalent fuel energy : Gain  Gain=Wbatt/100/0.95  SaturateOnIntegerOverflow=on  OutDataTypeStr=Inherit: Same as input  ParamDataTypeStr=Inherit: Same as input
  SOC*1 : Constant  Value=SOC_batt_start_value
  Saturation{1..4} (4 alike) : Saturate  UpperLimit=inf  LowerLimit=eps
  To Workspace : ToWorkspace  VariableName=FC  SampleTime=-1
  To Workspace1 : ToWorkspace  VariableName=DIST  SampleTime=-1
  To Workspace2 : ToWorkspace  VariableName=EC  SampleTime=-1
  "Ws -> Liter bensin" : Gain  Gain=1/Density  SaturateOnIntegerOverflow=on  OutDataTypeStr=Inherit: Same as input  ParamDataTypeStr=Inherit: Same as input
  "Ws -> Liter bensin1" : Gain  Gain=1/Density  SaturateOnIntegerOverflow=on  OutDataTypeStr=Inherit: Same as input  ParamDataTypeStr=Inherit: Same as input
  "Ws -> kWh" : Gain  Gain=1/3.6e6  SaturateOnIntegerOverflow=on  OutDataTypeStr=Inherit: Same as input  ParamDataTypeStr=Inherit: Same as input
  "meter -> mil" : Gain  Gain=1/10000  SaturateOnIntegerOverflow=on  OutDataTypeStr=Inherit: Same as input  ParamDataTypeStr=Inherit: Same as input
  v->s : Integrator  InitialCondition=100  LimitOutput=on  LowerSaturationLimit=100
  FC : Outport  VectorParamsAs1DForOutWhenUnconnected=off
  FCcomp : Outport  Port=2  VectorParamsAs1DForOutWhenUnconnected=off
  EC : Outport  Port=3  VectorParamsAs1DForOutWhenUnconnected=off
  dist (mil) : Outport  Port=4  VectorParamsAs1DForOutWhenUnconnected=off
  wires:
  "Ws -> Liter bensin"/1 -> -> L/mil/1
  v->s/1 -> "meter -> mil"/1
  -> L/mil/1 -> Saturation1/1
  Speed/1 -> v->s/1
  Saturation1/1 -> FC/1, To Workspace/1
  "meter -> mil"/1 -> -> L/mil1/2, -> kWh/mil/2, -> L/mil/2, dist (mil)/1, To Workspace1/1
  Fuel energy/1 -> Comp/2, "Ws -> Liter bensin"/1
  If EM is unable the ICE fills in1/1 -> SOC deviation equivalent fuel energy/1
  [EtaICEave] -> Saturation3/1
  Saturation2/1 -> FCcomp/1
  -> L/mil1/1 -> Saturation2/1
  "Ws -> Liter bensin1"/1 -> -> L/mil1/1
  Comp/1 -> "Ws -> Liter bensin1"/1
  SOC deviation equivalent fuel energy/1 -> Product1/1, "Ws -> kWh"/1
  Product1/1 -> Comp/1
  -> kWh/mil/1 -> Saturation4/1
  Saturation4/1 -> To Workspace2/1, EC/1
  "Ws -> kWh"/1 -> -> kWh/mil/1
  Saturation3/1 -> Product1/2
  SOC*1/1 -> If EM is unable the ICE fills in1/1
  [SOC] -> If EM is unable the ICE fills in1/2

== system Parallel/spdref ==
  Cycle : Scope  NumInputPorts=5
  Demux : Demux  Outputs=5
  Flat : Constant  Value=0
  Gain1 : Gain  Gain=1/1000  SaturateOnIntegerOverflow=on  OutDataTypeStr=Inherit: Same as input  ParamDataTypeStr=Inherit: Same as input
  Gain2 : Gain  Gain=3.6  SaturateOnIntegerOverflow=on  OutDataTypeStr=Inherit: Same as input  ParamDataTypeStr=Inherit: Same as input
  Gain3 : Gain  Gain=100  SaturateOnIntegerOverflow=on  OutDataTypeStr=Inherit: Same as input  ParamDataTypeStr=Inherit: Same as input
  Manual Switch : ManualSwitch
  Switch : Switch  Threshold=0.50
  Switch1 : Switch  Threshold=0.5
  Trigonometric Function : Trigonometry
  Variation : Constant
  v-buss2 : FromWorkspace  VariableName=cycle  SampleTime=.2  ZeroCross=off
  Speed ref : Outport  VectorParamsAs1DForOutWhenUnconnected=off
  tag scope: Altitude=global, SlideInAvailable=global, Slope=global
  wires:
  v-buss2/1 -> Demux/1
  Demux/4 -> Switch1/1
  Demux/3 -> Switch/1
  Demux/2 -> Gain1/1
  Flat/1 -> Switch1/3, Switch/3, Manual Switch/2
  Switch/1 -> Cycle/3, [Altitude]
  Switch1/1 -> Trigonometric Function/1, [Slope]
  Variation/1 -> Manual Switch/1
  Manual Switch/1 -> Switch/2, Switch1/2
  Gain1/1 -> Cycle/2
  Gain2/1 -> Cycle/1
  Demux/5 -> Cycle/5, [SlideInAvailable]
  Demux/1 -> Gain2/1, Speed ref/1
  Gain3/1 -> Cycle/4
  Trigonometric Function/1 -> Gain3/1

== system Parallel/Battery/- Chemical Power ==
  Pterm : Inport
  Look-Up Table : Lookup  InputValues=Pbatt  Table=EtaBATT  SaturateOnIntegerOverflow=on
  P/ n : Product  Inputs=**  InputSameDT=on  SaturateOnIntegerOverflow=on  OutDataTypeStr=Inherit: Same as first input
  Saturation : Saturate  UpperLimit=max(Pbatt)  LowerLimit=min(Pbatt)
  Pcharge : Outport  InitialOutput=0  VectorParamsAs1DForOutWhenUnconnected=off
  eta : Outport  Port=2  InitialOutput=0  VectorParamsAs1DForOutWhenUnconnected=off
  wires:
  Pterm/1 -> P/ n/1, Saturation/1
  Saturation/1 -> Look-Up Table/1
  P/ n/1 -> Pcharge/1
  Look-Up Table/1 -> P/ n/2, eta/1

== system Parallel/Battery/Subsystem ==
  "Pcharge " : Inport
  Constant : Constant  Value=SOC_batt_ref_value/100*Wbatt
  Gain3 : Gain  Gain=100/Wbatt  SaturateOnIntegerOverflow=on  OutDataTypeStr=Inherit: Same as input  ParamDataTypeStr=Inherit: Same as input
  Ptrm1 : Sum  Inputs=+-  InputSameDT=on  SaturateOnIntegerOverflow=on  OutDataTypeStr=Inherit: Same as first input
  Saturation : Saturate  UpperLimit=100  LowerLimit=0
  W batt starts at 70% : Integrator  InitialCondition=SOC_batt_ref_value/100*Wbatt  LimitOutput=on  UpperSaturationLimit=1.2*Wbatt  LowerSaturationLimit=0
  W batt in [%] : Outport  VectorParamsAs1DForOutWhenUnconnected=off
  DeltaWbatt in [Ws] : Outport  Port=2  VectorParamsAs1DForOutWhenUnconnected=off
  wires:
  Gain3/1 -> Saturation/1
  W batt starts at 70%/1 -> Gain3/1, Ptrm1/1
  Saturation/1 -> W batt in [%]/1
  Constant/1 -> Ptrm1/2
  Ptrm1/1 -> DeltaWbatt in [Ws]/1
  "Pcharge "/1 -> W batt starts at 70%/1

== system Parallel/Electric Machine model/Look-Up Table (2-D) ==
  Rows : Inport
  Cols : Inport  Port=2
  Look-Up Table (2-D) : Lookup2D  RowIndex=x  ColumnIndex=y  Table=t  SaturateOnIntegerOverflow=on  InputSameDT=on
  Out1 : Outport  VectorParamsAs1DForOutWhenUnconnected=off
  wires:
  Rows/1 -> Look-Up Table (2-D)/1
  Cols/1 -> Look-Up Table (2-D)/2
  Look-Up Table (2-D)/1 -> Out1/1

== system Parallel/Electric Machine model/Medelvärde ==
  note: Denna del "mäter" tiden då motorn
      | är till, d.v.s. då verkningsgraden är
      | större än 1 %. Om den är 5 % antas
      | motorn stå still.
  In : Inport
  Integral : Integrator
  Integral1 : Integrator  InitialCondition=eps  LimitOutput=on  LowerSaturationLimit=eps
  Medelv : Product  Inputs=*/  InputSameDT=on  SaturateOnIntegerOverflow=on  OutDataTypeStr=Inherit: Same as first input
  Medelv1 : Product  Inputs=**  InputSameDT=on  SaturateOnIntegerOverflow=on  OutDataTypeStr=Inherit: Same as first input
  Mux : Mux  Inputs=2
  Relay : Relay  OnSwitchValue=0.05  OffSwitchValue=0.04
  "Inst, Ave" : Outport  VectorParamsAs1DForOutWhenUnconnected=off
  wires:
  Integral1/1 -> Medelv/2
  Integral/1 -> Medelv/1
  In/1 -> Relay/1, Mux/1, Medelv1/1
  Relay/1 -> Integral1/1, Medelv1/2
  Medelv/1 -> Mux/2
  Mux/1 -> "Inst, Ave"/1
  Medelv1/1 -> Integral/1

== system Parallel/Electric Machine model/Subsystem ==
  T : Inport
  w : Inport  Port=2
  Abs2 : Abs  SaturateOnIntegerOverflow=on
  Constant : Constant  Value=eps
  EM torque1 : Product  Inputs=/*  InputSameDT=on  SaturateOnIntegerOverflow=on  OutDataTypeStr=Inherit: Same as first input
  T*w_ice : Product  Inputs=**  InputSameDT=on  SaturateOnIntegerOverflow=on  OutDataTypeStr=Inherit: Same as first input
  maxP : Saturate  UpperLimit=Pmax  LowerLimit=-Pmax
  maxT : Saturate  UpperLimit=Tmax  LowerLimit=-Tmax
  not div by 0 : Sum  InputSameDT=on  SaturateOnIntegerOverflow=on  OutDataTypeStr=Inherit: Same as first input
  Tlim : Outport  VectorParamsAs1DForOutWhenUnconnected=off
  wires:
  w/1 -> Abs2/1
  T/1 -> T*w_ice/2
  T*w_ice/1 -> maxP/1
  Abs2/1 -> not div by 0/2
  Constant/1 -> not div by 0/1
  maxP/1 -> EM torque1/2
  EM torque1/1 -> maxT/1
  not div by 0/1 -> EM torque1/1, T*w_ice/1
  maxT/1 -> Tlim/1

== system Parallel/ICE-model/FuelPower ==
  Rows : Inport
  Cols : Inport  Port=2
  Look-Up Table (2-D) : Lookup2D  RowIndex=x  ColumnIndex=y  Table=t  SaturateOnIntegerOverflow=on  InputSameDT=on
  Out1 : Outport  VectorParamsAs1DForOutWhenUnconnected=off
  wires:
  Look-Up Table (2-D)/1 -> Out1/1
  Cols/1 -> Look-Up Table (2-D)/2
  Rows/1 -> Look-Up Table (2-D)/1

== system Parallel/ICE-model/Generator load ==
  ICE speed : Inport
  Constant : Constant  Value=Paux
  Generator Efficiency : Constant  Value=Eta_gen
  Generator Mech Power : Product  Inputs=/*  InputSameDT=on  SaturateOnIntegerOverflow=on  OutDataTypeStr=Inherit: Same as first input
  Generator Mech Torque : Product  Inputs=/*  InputSameDT=on  SaturateOnIntegerOverflow=on  OutDataTypeStr=Inherit: Same as first input
  Saturation : Saturate  UpperLimit=Paux*2/(wice_max/5)  LowerLimit=0
  Generator torque : Outport  VectorParamsAs1DForOutWhenUnconnected=off
  wires:
  Constant/1 -> Generator Mech Power/2
  Generator Efficiency/1 -> Generator Mech Power/1
  Generator Mech Power/1 -> Generator Mech Torque/2
  ICE speed/1 -> Generator Mech Torque/1
  Generator Mech Torque/1 -> Saturation/1
  Saturation/1 -> Generator torque/1

== system Parallel/ICE-model/ICE efficiency ==
  Rows : Inport
  Cols : Inport  Port=2
  Look-Up Table (2-D) : Lookup2D  RowIndex=x  ColumnIndex=y  Table=t  SaturateOnIntegerOverflow=on  InputSameDT=on
  Out1 : Outport  VectorParamsAs1DForOutWhenUnconnected=off
  wires:
  Look-Up Table (2-D)/1 -> Out1/1
  Cols/1 -> Look-Up Table (2-D)/2
  Rows/1 -> Look-Up Table (2-D)/1

== system Parallel/ICE-model/Medelvärde ==
  note: Denna del "mäter" tiden då motorn
      | är till, d.v.s. då verkningsgraden är
      | större än 1 %. Om den är 5 % antas
      | motorn stå still.
  In : Inport
  In1 : Inport  Port=2
  Integral : Integrator  InitialCondition=0.145
  Integral1 : Integrator  InitialCondition=4  LimitOutput=on  LowerSaturationLimit=1
  Medelv : Product  Inputs=*/  InputSameDT=on  SaturateOnIntegerOverflow=on  OutDataTypeStr=Inherit: Same as first input
  Medelv1 : Product  Inputs=**  InputSameDT=on  SaturateOnIntegerOverflow=on  OutDataTypeStr=Inherit: Same as first input
  Mux : Mux  Inputs=2
  Mux1 : Mux  Inputs=2
  Relay : Relay  OnSwitchValue=0.15  OffSwitchValue=0.14
  Scope : Scope
  "Inst, Ave" : Outport  VectorParamsAs1DForOutWhenUnconnected=off
  wires:
  Mux/1 -> "Inst, Ave"/1
  Medelv/1 -> Mux/2, Mux1/1
  Relay/1 -> Integral1/1, Medelv1/2
  In/1 -> Relay/1, Medelv1/1, Mux/1
  Integral/1 -> Medelv/1
  Integral1/1 -> Medelv/2
  Medelv1/1 -> Integral/1
  Mux1/1 -> Scope/1
  In1/1 -> Mux1/2

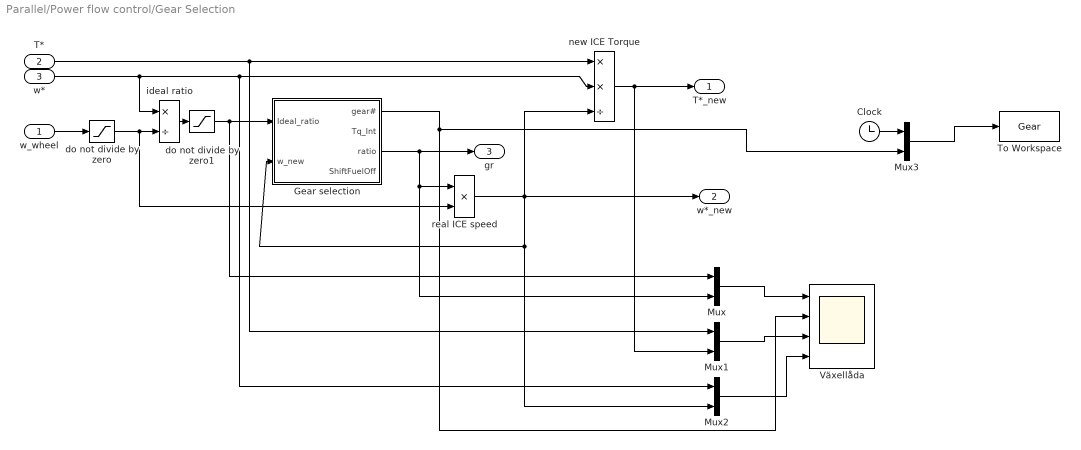
== system Parallel/Power flow control/Gear Selection ==
  w_wheel : Inport
  T* : Inport  Port=2
  w* : Inport  Port=3
  Clock : Clock
  Gear selection : Subsystem
  Mux{,1..3} (4 alike) : Mux  Inputs=2
  To Workspace : ToWorkspace  VariableName=Gear  SampleTime=-1
  Växellåda : Scope  NumInputPorts=4
  do not divide by zero : Saturate  UpperLimit=inf  LowerLimit=wice_min/utvx_max
  do not divide by zero1 : Saturate  UpperLimit=1.2*max(Utvx_vect)  LowerLimit=eps
  ideal ratio : Product  Inputs=*/  InputSameDT=on  SaturateOnIntegerOverflow=on  OutDataTypeStr=Inherit: Same as first input
  new ICE Torque : Product  Inputs=**/  InputSameDT=on  SaturateOnIntegerOverflow=on  OutDataTypeStr=Inherit: Same as first input
  real ICE speed : Product  Inputs=**  InputSameDT=on  SaturateOnIntegerOverflow=on  OutDataTypeStr=Inherit: Same as first input
  T*_new : Outport  VectorParamsAs1DForOutWhenUnconnected=off
  w*_new : Outport  Port=2  VectorParamsAs1DForOutWhenUnconnected=off
  gr : Outport  Port=3  VectorParamsAs1DForOutWhenUnconnected=off
  wires:
  w*/1 -> ideal ratio/1, Mux2/1, new ICE Torque/2
  ideal ratio/1 -> do not divide by zero1/1
  real ICE speed/1 -> w*_new/1, new ICE Torque/3, Mux2/2, Gear selection/2(w_new)
  T*/1 -> Mux1/1, new ICE Torque/1
  do not divide by zero/1 -> ideal ratio/2, real ICE speed/2
  w_wheel/1 -> do not divide by zero/1
  Mux/1 -> Växellåda/1
  Mux1/1 -> Växellåda/3
  Mux2/1 -> Växellåda/4
  Gear selection/3(ratio) -> real ICE speed/1, Mux/2, gr/1
  Gear selection/1(gear#) -> Mux3/2, Växellåda/2
  new ICE Torque/1 -> Mux1/2, T*_new/1
  do not divide by zero1/1 -> Gear selection/1(Ideal_ratio), Mux/1
  Clock/1 -> Mux3/1
  Mux3/1 -> To Workspace/1

== system Parallel/Power flow control/Laddnings-reglering ==
  SOC : Inport
  10% avvikelse ger 10 kW motoreffekt : Gain  Gain=ksoc/4  OutDataTypeStr=Inherit: Same as input  ParamDataTypeStr=Inherit: Same as input
  Abs : Abs  SaturateOnIntegerOverflow=on
  Look-Up Table : Lookup  InputValues=[-15:1:15]  Table=ksoc_vect  SaturateOnIntegerOverflow=on
  Manual Switch : ManualSwitch  CurrentSetting=0
  Mux : Mux  Inputs=2
  Product : Product  SaturateOnIntegerOverflow=on  OutDataTypeStr=Inherit: Same as first input
  SOC* : Constant  Value=SOC_batt_ref_value
  Scope : Scope  NumInputPorts=2
  Sum1 : Sum  Inputs=-+  InputSameDT=on  SaturateOnIntegerOverflow=on  OutDataTypeStr=Inherit: Same as first input
  P charge * : Outport  InitialOutput=0  VectorParamsAs1DForOutWhenUnconnected=off
  wires:
  SOC*/1 -> Sum1/2
  Sum1/1 -> 10% avvikelse ger 10 kW motoreffekt/1, Abs/1, Look-Up Table/1
  SOC/1 -> Sum1/1
  Look-Up Table/1 -> Product/1
  10% avvikelse ger 10 kW motoreffekt/1 -> Manual Switch/1, Mux/1
  Product/1 -> Manual Switch/2, Mux/2
  Mux/1 -> Scope/1
  Abs/1 -> Product/2, Scope/2
  Manual Switch/1 -> P charge */1

== system Parallel/Power flow control/Optimal operating point ==
  Pice* : Inport
  -> w1 : Product  Inputs=**  InputSameDT=on  SaturateOnIntegerOverflow=on  OutDataTypeStr=Inherit: Same as first input
  LP-filter : Subsystem
  NO ICE Torque @ to low efficiency : Relay  OnSwitchValue=0.25  OffSwitchValue=0.22
  Saturation1 : Saturate  UpperLimit=inf  LowerLimit=eps
  Saturation2 : Saturate  UpperLimit=Pice_max  LowerLimit=eps
  Saturation3 : Saturate  UpperLimit=Tice_max  LowerLimit=eps
  Saturation4 : Saturate  UpperLimit=wice_max  LowerLimit=wice_min
  Topt_ice : Lookup  InputValues=PtoT(:,1)  Table=PtoT(:,2)  LookUpMeth=Interpolation-Use End Values  SaturateOnIntegerOverflow=on
  Wopt_ice : Lookup  InputValues=PtoT(:,1)  Table=PtoT(:,4)  LookUpMeth=Interpolation-Use End Values  SaturateOnIntegerOverflow=on
  eta_ice : Lookup  InputValues=PtoT(:,1)  Table=PtoT(:,3)  SaturateOnIntegerOverflow=on
  IceOff : Outport  InitialOutput=0  VectorParamsAs1DForOutWhenUnconnected=off
  T* : Outport  Port=2  InitialOutput=0  VectorParamsAs1DForOutWhenUnconnected=off
  w* : Outport  Port=3  InitialOutput=0  VectorParamsAs1DForOutWhenUnconnected=off
  eta : Outport  Port=4  InitialOutput=0  VectorParamsAs1DForOutWhenUnconnected=off
  wires:
  Pice*/1 -> Saturation1/1
  Topt_ice/1 -> Saturation3/1
  eta_ice/1 -> eta/1, NO ICE Torque @ to low efficiency/1
  Saturation1/1 -> LP-filter/1(P ice*)
  Saturation3/1 -> -> w1/1
  Saturation2/1 -> Wopt_ice/1, eta_ice/1, Topt_ice/1
  LP-filter/1(P ice) -> Saturation2/1
  Wopt_ice/1 -> Saturation4/1
  Saturation4/1 -> w*/1
  -> w1/1 -> T*/1
  NO ICE Torque @ to low efficiency/1 -> IceOff/1, -> w1/2
